simulink model "apartado233"  (Simulink 7.1)
settings: Solver=ode45  StartTime=0.0  StopTime=10000  RelTol=1e-3
undefined symbols (not defined in the file): p
libraries: simeventsrouting1 x15, simeventssink1 x13, simeventsattributes2 x6, simeventsqueue1 x6, simeventsgates1 x6, simeventsgenerators1 x6, simeventstiming1 x4, simeventsserver1 x3
settings Model: Creator=EmP  LastModifiedBy=EmP
settings SimEventsCC: propLogEventsScheduled=0  propLogEventsExecuted=0  propLogDepartureEvents=0  propDisplayEventCalendar=0  propDiagAttribOutput=1  propDiagFcnCallOutput=1  propDiagStatOutput=0

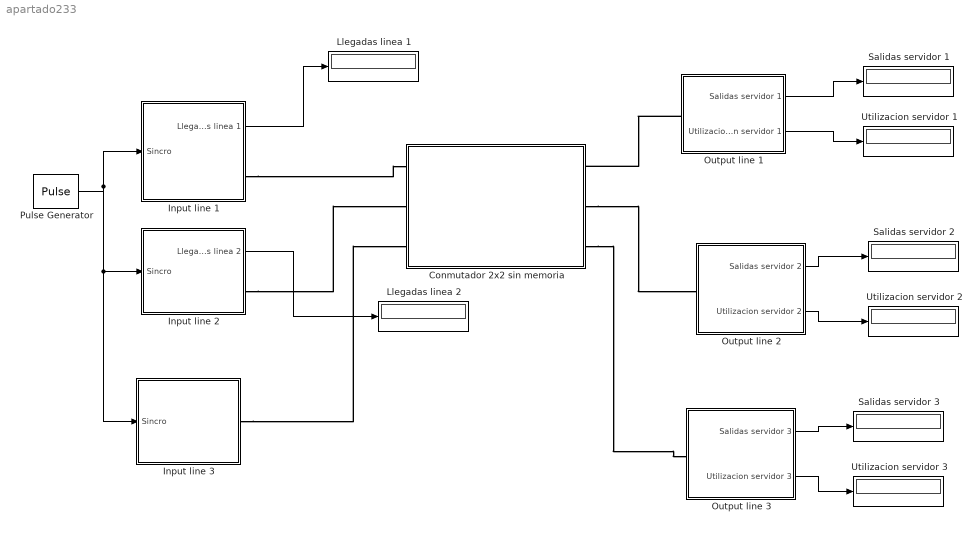
== system apartado233 ==
  Conmutador 2x2 sin memoria : Subsystem
  Input line 1 : Subsystem
  Input line 2 : Subsystem
  Input line 3 : Subsystem
  Llegadas linea 1 : Display
  Llegadas linea 2 : Display
  Output line 1 : Subsystem
  Output line 2 : Subsystem
  Output line 3 : Subsystem
  Pulse Generator : DiscretePulseGenerator  PulseType=Time based  Period=1  PulseWidth=50
  Salidas servidor 1 : Display
  Salidas servidor 2 : Display
  Salidas servidor 3 : Display
  Utilizacion servidor 1 : Display
  Utilizacion servidor 2 : Display
  Utilizacion servidor 3 : Display
  wires:
  Pulse Generator/1 -> Input line 1/1(Sincro), Input line 2/1(Sincro), Input line 3/1(Sincro)
  Input line 1/1(Llegadas linea 1) -> Llegadas linea 1/1
  Input line 2/1(Llegadas linea 2) -> Llegadas linea 2/1
  Output line 1/2(Utilizacion servidor 1) -> Utilizacion servidor 1/1
  Output line 1/1(Salidas servidor 1) -> Salidas servidor 1/1
  Output line 2/1(Salidas servidor 2) -> Salidas servidor 2/1
  Output line 2/2(Utilizacion servidor 2) -> Utilizacion servidor 2/1
  Output line 3/1(Salidas servidor 3) -> Salidas servidor 3/1
  Output line 3/2(Utilizacion servidor 3) -> Utilizacion servidor 3/1
  connections:
  Input line 1/RConn1 -- Conmutador 2x2 sin memoria/LConn1
  Input line 2/RConn1 -- Conmutador 2x2 sin memoria/LConn2
  Output line 1/LConn1 -- Conmutador 2x2 sin memoria/RConn1
  Conmutador 2x2 sin memoria/RConn2 -- Output line 2/LConn1
  Input line 3/RConn1 -- Conmutador 2x2 sin memoria/LConn3
  Conmutador 2x2 sin memoria/RConn3 -- Output line 3/LConn1

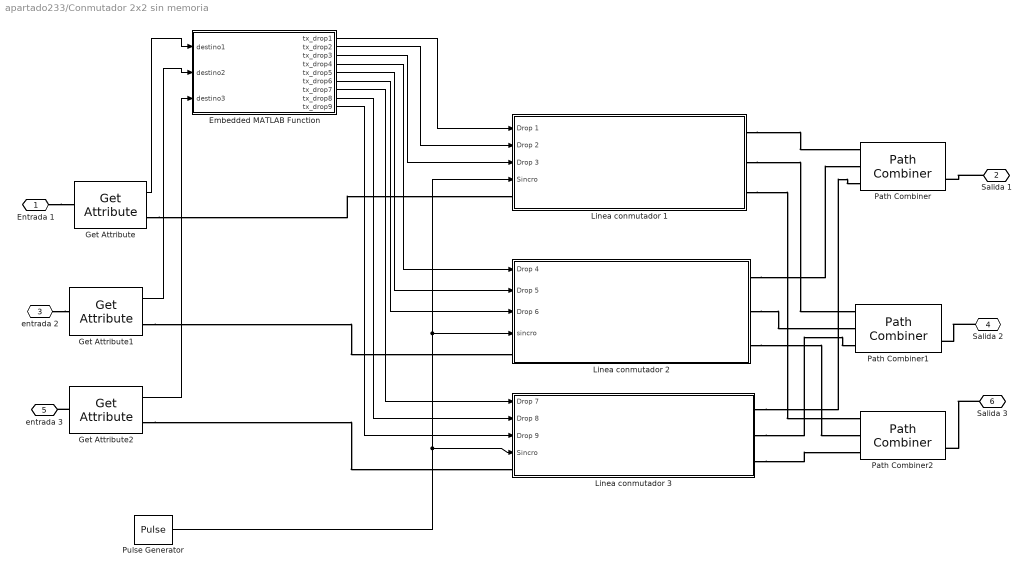
== system apartado233/Conmutador 2x2 sin memoria ==
  Embedded MATLAB Function : Stateflow chart
  Get Attribute : simeventsattributes2/Get Attribute  Priority=1  DialogController=des_ddg_create  DialogControllerArgs=DataTag1  SystemSampleTime=-1  AttributeName=Destino1  AttributeMissing=Error  AttributeDefaultValue=1  AttributeSendTiming=After entity departure  AttributeTreatAsVector=1  StatNumberDeparted=Off  EvaluatedDefaultAttributeValue={[]}
  Get Attribute1 : simeventsattributes2/Get Attribute  Priority=1  DialogController=des_ddg_create  DialogControllerArgs=DataTag3  SystemSampleTime=-1  AttributeName=Destino2  AttributeMissing=Error  AttributeDefaultValue=1  AttributeSendTiming=After entity departure  AttributeTreatAsVector=1  StatNumberDeparted=Off  EvaluatedDefaultAttributeValue={[]}
  Get Attribute2 : simeventsattributes2/Get Attribute  Priority=1  DialogController=des_ddg_create  DialogControllerArgs=DataTag5  SystemSampleTime=-1  AttributeName=Destino3  AttributeMissing=Error  AttributeDefaultValue=1  AttributeSendTiming=After entity departure  AttributeTreatAsVector=1  StatNumberDeparted=Off  EvaluatedDefaultAttributeValue={[]}
  Linea conmutador 1 : Subsystem
  Linea conmutador 2 : Subsystem
  Linea conmutador 3 : Subsystem
  Path Combiner : simeventsrouting1/Path Combiner  Priority=1  SystemSampleTime=-1  NumberInputPorts=3  InputPortPrecedence=IN1 port  InitialSeed=45675  SpecifyEventPriority=off  PriorityPathCombinerPortPrecedenceSelection=4100  StatNumberDeparted=On  StatLastArrivalPort=Off  EvaluatedNumPorts=3
  Path Combiner1 : simeventsrouting1/Path Combiner  Priority=1  SystemSampleTime=-1  NumberInputPorts=3  InputPortPrecedence=IN1 port  InitialSeed=45675  SpecifyEventPriority=off  PriorityPathCombinerPortPrecedenceSelection=4100  StatNumberDeparted=On  StatLastArrivalPort=Off  EvaluatedNumPorts=3
  Path Combiner2 : simeventsrouting1/Path Combiner  Priority=1  SystemSampleTime=-1  NumberInputPorts=3  InputPortPrecedence=IN1 port  InitialSeed=45675  SpecifyEventPriority=off  PriorityPathCombinerPortPrecedenceSelection=4100  StatNumberDeparted=On  StatLastArrivalPort=Off  EvaluatedNumPorts=3
  Pulse Generator : DiscretePulseGenerator  PulseType=Time based  Period=1  PulseWidth=50  PhaseDelay=0.5
  Entrada 1 : PMIOPort  Port=1  Side=Left
  Salida 1 : PMIOPort  Orientation=left  Port=2  Side=Right
  entrada 2 : PMIOPort  Port=3  Side=Left
  Salida 2 : PMIOPort  Orientation=left  Port=4  Side=Right
  entrada 3 : PMIOPort  Port=5  Side=Left
  Salida 3 : PMIOPort  Orientation=left  Port=6  Side=Right
  wires:
  Pulse Generator/1 -> Linea conmutador 3/4(Sincro), Linea conmutador 2/4(sincro), Linea conmutador 1/4(Sincro)
  Embedded MATLAB Function/1(tx_drop1) -> Linea conmutador 1/1(Drop 1)
  Embedded MATLAB Function/2(tx_drop2) -> Linea conmutador 1/2(Drop 2)
  Embedded MATLAB Function/3(tx_drop3) -> Linea conmutador 1/3(Drop 3)
  Embedded MATLAB Function/4(tx_drop4) -> Linea conmutador 2/1(Drop 4)
  Embedded MATLAB Function/5(tx_drop5) -> Linea conmutador 2/2(Drop 5)
  Embedded MATLAB Function/6(tx_drop6) -> Linea conmutador 2/3(Drop 6)
  Embedded MATLAB Function/7(tx_drop7) -> Linea conmutador 3/1(Drop 7)
  Embedded MATLAB Function/8(tx_drop8) -> Linea conmutador 3/2(Drop 8)
  Embedded MATLAB Function/9(tx_drop9) -> Linea conmutador 3/3(Drop 9)
  Get Attribute/1 -> Embedded MATLAB Function/1(destino1)
  Get Attribute1/1 -> Embedded MATLAB Function/2(destino2)
  Get Attribute2/1 -> Embedded MATLAB Function/3(destino3)
  connections:
  Entrada 1/RConn1 -- Get Attribute/LConn1
  Salida 1/RConn1 -- Path Combiner/RConn1
  entrada 2/RConn1 -- Get Attribute1/LConn1
  Salida 2/RConn1 -- Path Combiner1/RConn1
  Salida 3/RConn1 -- Path Combiner2/RConn1
  Get Attribute2/LConn1 -- entrada 3/RConn1
  Get Attribute/RConn1 -- Linea conmutador 1/LConn1
  Get Attribute1/RConn1 -- Linea conmutador 2/LConn1
  Get Attribute2/RConn1 -- Linea conmutador 3/LConn1
  Linea conmutador 1/RConn1 -- Path Combiner/LConn1
  Linea conmutador 1/RConn2 -- Path Combiner1/LConn1
  Linea conmutador 1/RConn3 -- Path Combiner2/LConn1
  Linea conmutador 2/RConn1 -- Path Combiner/LConn2
  Linea conmutador 2/RConn2 -- Path Combiner1/LConn2
  Linea conmutador 2/RConn3 -- Path Combiner2/LConn2
  Linea conmutador 3/RConn1 -- Path Combiner/LConn3
  Linea conmutador 3/RConn2 -- Path Combiner1/LConn3
  Linea conmutador 3/RConn3 -- Path Combiner2/LConn3

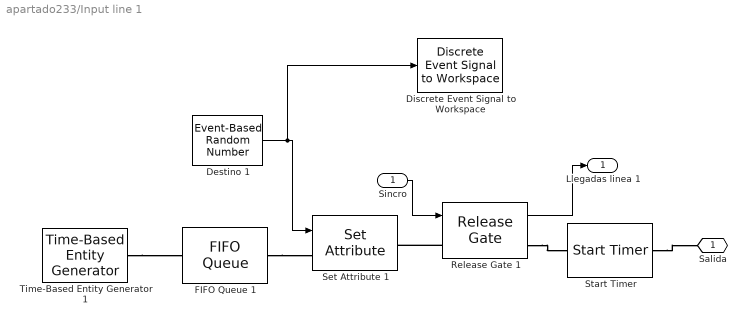
== system apartado233/Input line 1 ==
  Sincro : Inport
  Destino 1 : simeventsgenerators1/Signal Generators/Event-Based Random Number  SystemSampleTime=-1  distribution=Arbitrary discrete  meanExp=1  minUnif=1  maxUnif=2  pOneBern=0.25  pSuccessBino=0.5  numTrialBino=1  meanNorm=0  stdNorm=1  minTri=1  maxTri=3  modeTri=2  thresholdLogn=0  scaleLogn=1  shapeLogn=1  pSuccessGeo=0.5  meanPoiss=1  thresholdLogl=0  scaleLogl=1  thresholdGam=0  scaleGam=1  shapeGam=1  minBeta=0  maxBeta=1  shape1Beta=1  shape2Beta=1  minUnid=1  maxUnid=2  numValueUnid=2  thresholdWbl=0  scaleWbl=1  shapeWbl=1  valueVecCont=[0 1]  cdfVecCont=[0 1]  valueVecDisc=[0 1 2]  probVecDisc=[(1-p) p/2 p/2]  seed=875632  IsProcessed=on  isConnected=1
  Discrete Event Signal to Workspace : simeventssink1/Discrete Event Signal to Workspace  SystemSampleTime=-1  VariableName=destinoslinea1  SaveFormat=Array  IsMonitorOnly=off
  FIFO Queue 1 : simeventsqueue1/FIFO Queue  Priority=1  SystemSampleTime=-1  Capacity=inf  EnableTOPort=off  StatNumberDeparted=Off  StatNumberInBlock=Off  StatPendingEntity=Off  StatAverageWait=Off  StatAverageQueueLength=Off  StatNumberTimedout=Off
  Release Gate 1 : simeventsgates1/Release Gate  Priority=1  SystemSampleTime=-1  OpenGateUpon=Change in signal from port vc  SignalEdgeOption=Rising  SpecifyEventPriority=off  PriorityGateRelease=2200  StatNumberDeparted=On
  Set Attribute 1 : simeventsattributes2/Set Attribute  Priority=1  DialogController=des_ddg_create  DialogControllerArgs=DataTag39  SystemSampleTime=-1  AttributeFrom=Signal port  AttributeName=Destino1  AttributeTreatAsVector=1  AttributeValue=1  AttributeCreate=on  StatNumberDeparted=Off  EvaluatedAttributeValue={[]}
  Start Timer : simeventstiming1/Start Timer  Priority=0  SystemSampleTime=-1  TimerTag=retardo  TimerStartedOption=Warn and continue  StatNumberDeparted=Off
  Time-Based Entity Generator 1 : simeventsgenerators1/Entity Generators/Time-Based Entity Generator  Priority=1  DialogController=des_ddg_create  DialogControllerArgs=DataTag42  SystemSampleTime=-1  GenerateEntitiesUpon=Intergeneration time from dialog  Distribution=Constant  Minimum=0  Maximum=1  Mean=1  InitialSeed=12345  Period=0.5  PriorityEntityGeneration=300  GenerateEntityAtSimulationStart=on  ResponseWhenBlocked=Pause generation  ResponseWhenUnblocked=Immediate restart  EntityType=Blank  StatNumberDeparted=Off  StatPendingEntity=Off  StatAverageIntergenerationTime=Off
  Salida : PMIOPort  Orientation=left  Port=1  Side=Right
  Llegadas linea 1 : Outport  OutDataType=sfix(16)  OutScaling=2^0
  wires:
  Destino 1/1 -> Set Attribute 1/1, Discrete Event Signal to Workspace/1
  Sincro/1 -> Release Gate 1/1
  Release Gate 1/1 -> Llegadas linea 1/1
  connections:
  Time-Based Entity Generator 1/RConn1 -- FIFO Queue 1/LConn1
  FIFO Queue 1/RConn1 -- Set Attribute 1/LConn1
  Release Gate 1/LConn1 -- Set Attribute 1/RConn1
  Start Timer/RConn1 -- Salida/RConn1
  Release Gate 1/RConn1 -- Start Timer/LConn1

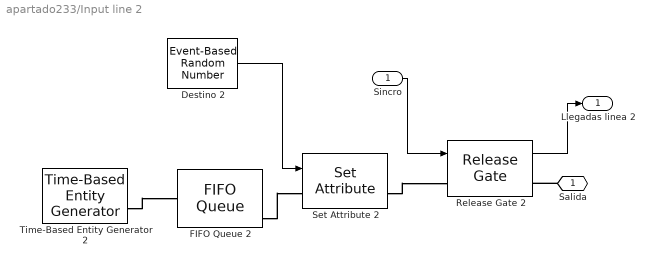
== system apartado233/Input line 2 ==
  Sincro : Inport
  Destino 2 : simeventsgenerators1/Signal Generators/Event-Based Random Number  SystemSampleTime=-1  distribution=Arbitrary discrete  meanExp=1  minUnif=1  maxUnif=1  pOneBern=0.25  pSuccessBino=0.5  numTrialBino=1  meanNorm=0  stdNorm=1  minTri=1  maxTri=3  modeTri=2  thresholdLogn=0  scaleLogn=1  shapeLogn=1  pSuccessGeo=0.5  meanPoiss=1  thresholdLogl=0  scaleLogl=1  thresholdGam=0  scaleGam=1  shapeGam=1  minBeta=0  maxBeta=1  shape1Beta=1  shape2Beta=1  minUnid=1  maxUnid=2  numValueUnid=2  thresholdWbl=0  scaleWbl=1  shapeWbl=1  valueVecCont=[0 1]  cdfVecCont=[0 1]  valueVecDisc=[0 1 2]  probVecDisc=[(1-p) p/2 p/2]  seed=0964  IsProcessed=on  isConnected=1
  FIFO Queue 2 : simeventsqueue1/FIFO Queue  Priority=1  SystemSampleTime=-1  Capacity=1000000  EnableTOPort=off  StatNumberDeparted=On  StatNumberInBlock=On  StatPendingEntity=Off  StatAverageWait=Off  StatAverageQueueLength=Off  StatNumberTimedout=Off
  Release Gate 2 : simeventsgates1/Release Gate  Priority=1  SystemSampleTime=-1  OpenGateUpon=Change in signal from port vc  SignalEdgeOption=Rising  SpecifyEventPriority=off  PriorityGateRelease=2200  StatNumberDeparted=On
  Set Attribute 2 : simeventsattributes2/Set Attribute  Priority=1  DialogController=des_ddg_create  DialogControllerArgs=DataTag46  SystemSampleTime=-1  AttributeFrom=Signal port  AttributeName=Destino2  AttributeTreatAsVector=1  AttributeValue=1  AttributeCreate=on  StatNumberDeparted=On  EvaluatedAttributeValue={[]}
  Time-Based Entity Generator 2 : simeventsgenerators1/Entity Generators/Time-Based Entity Generator  Priority=1  DialogController=des_ddg_create  DialogControllerArgs=DataTag48  SystemSampleTime=-1  GenerateEntitiesUpon=Intergeneration time from dialog  Distribution=Constant  Minimum=0  Maximum=1  Mean=1  InitialSeed=543541  Period=1  PriorityEntityGeneration=300  GenerateEntityAtSimulationStart=on  ResponseWhenBlocked=Pause generation  ResponseWhenUnblocked=Immediate restart  EntityType=Blank  StatNumberDeparted=On  StatPendingEntity=Off  StatAverageIntergenerationTime=Off
  Salida : PMIOPort  Orientation=left  Port=1  Side=Right
  Llegadas linea 2 : Outport  OutDataType=sfix(16)  OutScaling=2^0
  wires:
  Destino 2/1 -> Set Attribute 2/1
  Sincro/1 -> Release Gate 2/1
  Release Gate 2/1 -> Llegadas linea 2/1
  connections:
  Time-Based Entity Generator 2/RConn1 -- FIFO Queue 2/LConn1
  FIFO Queue 2/RConn1 -- Set Attribute 2/LConn1
  Set Attribute 2/RConn1 -- Release Gate 2/LConn1
  Salida/RConn1 -- Release Gate 2/RConn1

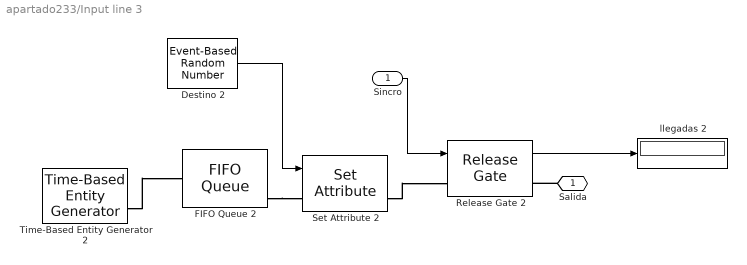
== system apartado233/Input line 3 ==
  Sincro : Inport
  Destino 2 : simeventsgenerators1/Signal Generators/Event-Based Random Number  SystemSampleTime=-1  distribution=Arbitrary discrete  meanExp=1  minUnif=1  maxUnif=1  pOneBern=0.25  pSuccessBino=0.5  numTrialBino=1  meanNorm=0  stdNorm=1  minTri=1  maxTri=3  modeTri=2  thresholdLogn=0  scaleLogn=1  shapeLogn=1  pSuccessGeo=0.5  meanPoiss=1  thresholdLogl=0  scaleLogl=1  thresholdGam=0  scaleGam=1  shapeGam=1  minBeta=0  maxBeta=1  shape1Beta=1  shape2Beta=1  minUnid=1  maxUnid=2  numValueUnid=2  thresholdWbl=0  scaleWbl=1  shapeWbl=1  valueVecCont=[0 1]  cdfVecCont=[0 1]  valueVecDisc=[0 1 2]  probVecDisc=[(1-p) p/2 p/2]  seed=45287634  IsProcessed=on  isConnected=1
  FIFO Queue 2 : simeventsqueue1/FIFO Queue  Priority=1  SystemSampleTime=-1  Capacity=1000000  EnableTOPort=off  StatNumberDeparted=On  StatNumberInBlock=On  StatPendingEntity=Off  StatAverageWait=Off  StatAverageQueueLength=Off  StatNumberTimedout=Off
  Release Gate 2 : simeventsgates1/Release Gate  Priority=1  SystemSampleTime=-1  OpenGateUpon=Change in signal from port vc  SignalEdgeOption=Rising  SpecifyEventPriority=off  PriorityGateRelease=2200  StatNumberDeparted=On
  Set Attribute 2 : simeventsattributes2/Set Attribute  Priority=1  DialogController=des_ddg_create  DialogControllerArgs=DataTag52  SystemSampleTime=-1  AttributeFrom=Signal port  AttributeName=Destino3  AttributeTreatAsVector=1  AttributeValue=1  AttributeCreate=on  StatNumberDeparted=On  EvaluatedAttributeValue={[]}
  Time-Based Entity Generator 2 : simeventsgenerators1/Entity Generators/Time-Based Entity Generator  Priority=1  DialogController=des_ddg_create  DialogControllerArgs=DataTag54  SystemSampleTime=-1  GenerateEntitiesUpon=Intergeneration time from dialog  Distribution=Constant  Minimum=0  Maximum=1  Mean=1  InitialSeed=543541  Period=1  PriorityEntityGeneration=300  GenerateEntityAtSimulationStart=on  ResponseWhenBlocked=Pause generation  ResponseWhenUnblocked=Immediate restart  EntityType=Blank  StatNumberDeparted=On  StatPendingEntity=Off  StatAverageIntergenerationTime=Off
  llegadas 2 : Display
  Salida : PMIOPort  Orientation=left  Port=1  Side=Right
  wires:
  Destino 2/1 -> Set Attribute 2/1
  Sincro/1 -> Release Gate 2/1
  Release Gate 2/1 -> llegadas 2/1
  connections:
  Time-Based Entity Generator 2/RConn1 -- FIFO Queue 2/LConn1
  FIFO Queue 2/RConn1 -- Set Attribute 2/LConn1
  Set Attribute 2/RConn1 -- Release Gate 2/LConn1
  Salida/RConn1 -- Release Gate 2/RConn1

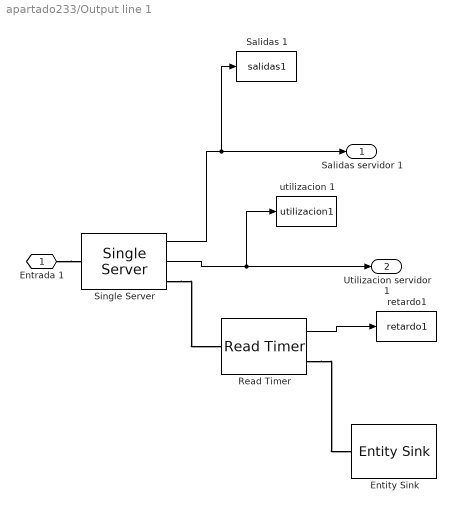
== system apartado233/Output line 1 ==
  Entity Sink : simeventssink1/Entity Sink  Priority=1  SystemSampleTime=-1  AvailableForArrivals=on  StatNumberArrived=Off
  Read Timer : simeventstiming1/Read Timer  Priority=0  SystemSampleTime=-1  TimerTag=retardo  TimerModeOption=Ignore  TimerStop=off  StatNumberDeparted=Off  StatTimerNumberDeparted=Off  StatTimeElapsed=Off  StatAverageTimeElapsed=On
  Salidas 1 : ToWorkspace  VariableName=salidas1  SampleTime=10000  SaveFormat=Array
  Single Server : simeventsserver1/Single Server  Priority=1  SystemSampleTime=-1  ServiceTimeFrom=Dialog  ServiceTime=0.99999  AttributeName=ServiceTime  PriorityServiceCompletion=500  PermitPreemption=off  SortingAttributeName=PriorityAttributeName  SortingDirection=Ascending  WriteToAttribute=off  ResidualAttributeName=ResidualServiceTime  CreateAttribute=on  EnableTOPort=off  StatNumberDeparted=On  StatNumberInBlock=Off  StatNumberPreempted=Off  StatPendingEntity=Off  StatAverageWait=Off  StatUtilization=On  StatNumberTimedout=Off
  retardo1 : ToWorkspace  VariableName=retardo1  SampleTime=10000  SaveFormat=Array
  utilizacion 1 : ToWorkspace  VariableName=utilizacion1  SampleTime=10000  SaveFormat=Array
  Entrada 1 : PMIOPort  Port=1  Side=Left
  Salidas servidor 1 : Outport  OutDataType=sfix(16)  OutScaling=2^0
  Utilizacion servidor 1 : Outport  Port=2  OutDataType=sfix(16)  OutScaling=2^0
  wires:
  Single Server/1 -> Salidas 1/1, Salidas servidor 1/1
  Single Server/2 -> Utilizacion servidor 1/1, utilizacion 1/1
  Read Timer/1 -> retardo1/1
  connections:
  Entrada 1/RConn1 -- Single Server/LConn1
  Read Timer/RConn1 -- Entity Sink/LConn1
  Single Server/RConn1 -- Read Timer/LConn1

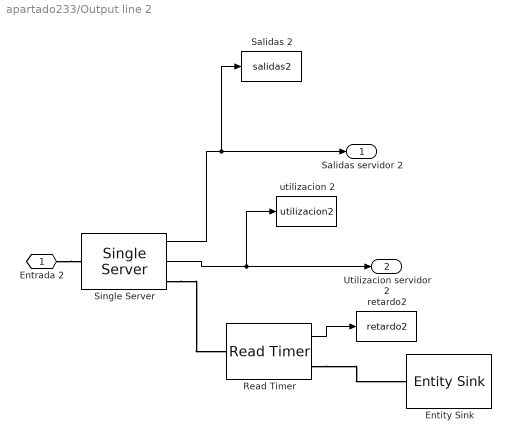
== system apartado233/Output line 2 ==
  Entity Sink : simeventssink1/Entity Sink  Priority=1  SystemSampleTime=-1  AvailableForArrivals=on  StatNumberArrived=Off
  Read Timer : simeventstiming1/Read Timer  Priority=0  SystemSampleTime=-1  TimerTag=retardo  TimerModeOption=Ignore  TimerStop=off  StatNumberDeparted=Off  StatTimerNumberDeparted=Off  StatTimeElapsed=Off  StatAverageTimeElapsed=On
  Salidas 2 : ToWorkspace  VariableName=salidas2  SampleTime=10000  SaveFormat=Array
  Single Server : simeventsserver1/Single Server  Priority=1  SystemSampleTime=-1  ServiceTimeFrom=Dialog  ServiceTime=0.99999  AttributeName=ServiceTime  PriorityServiceCompletion=500  PermitPreemption=off  SortingAttributeName=PriorityAttributeName  SortingDirection=Ascending  WriteToAttribute=off  ResidualAttributeName=ResidualServiceTime  CreateAttribute=on  EnableTOPort=off  StatNumberDeparted=On  StatNumberInBlock=Off  StatNumberPreempted=Off  StatPendingEntity=Off  StatAverageWait=Off  StatUtilization=On  StatNumberTimedout=Off
  retardo2 : ToWorkspace  VariableName=retardo2  SampleTime=10000  SaveFormat=Array
  utilizacion 2 : ToWorkspace  VariableName=utilizacion2  SampleTime=10000  SaveFormat=Array
  Entrada 2 : PMIOPort  Port=1  Side=Left
  Salidas servidor 2 : Outport  OutDataType=sfix(16)  OutScaling=2^0
  Utilizacion servidor 2 : Outport  Port=2  OutDataType=sfix(16)  OutScaling=2^0
  wires:
  Single Server/1 -> Salidas 2/1, Salidas servidor 2/1
  Single Server/2 -> Utilizacion servidor 2/1, utilizacion 2/1
  Read Timer/1 -> retardo2/1
  connections:
  Entrada 2/RConn1 -- Single Server/LConn1
  Read Timer/RConn1 -- Entity Sink/LConn1
  Single Server/RConn1 -- Read Timer/LConn1

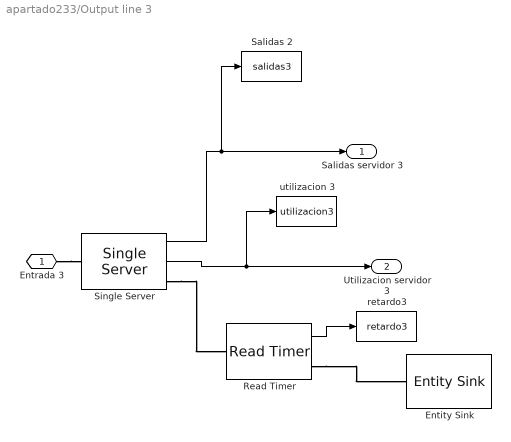
== system apartado233/Output line 3 ==
  Entity Sink : simeventssink1/Entity Sink  Priority=1  SystemSampleTime=-1  AvailableForArrivals=on  StatNumberArrived=Off
  Read Timer : simeventstiming1/Read Timer  Priority=0  SystemSampleTime=-1  TimerTag=retardo  TimerModeOption=Ignore  TimerStop=off  StatNumberDeparted=Off  StatTimerNumberDeparted=Off  StatTimeElapsed=Off  StatAverageTimeElapsed=On
  Salidas 2 : ToWorkspace  VariableName=salidas3  SampleTime=10000  SaveFormat=Array
  Single Server : simeventsserver1/Single Server  Priority=1  SystemSampleTime=-1  ServiceTimeFrom=Dialog  ServiceTime=0.99999  AttributeName=ServiceTime  PriorityServiceCompletion=500  PermitPreemption=off  SortingAttributeName=PriorityAttributeName  SortingDirection=Ascending  WriteToAttribute=off  ResidualAttributeName=ResidualServiceTime  CreateAttribute=on  EnableTOPort=off  StatNumberDeparted=On  StatNumberInBlock=Off  StatNumberPreempted=Off  StatPendingEntity=Off  StatAverageWait=Off  StatUtilization=On  StatNumberTimedout=Off
  retardo3 : ToWorkspace  VariableName=retardo3  SampleTime=10000  SaveFormat=Array
  utilizacion 3 : ToWorkspace  VariableName=utilizacion3  SampleTime=10000  SaveFormat=Array
  Entrada 3 : PMIOPort  Port=1  Side=Left
  Salidas servidor 3 : Outport  OutDataType=sfix(16)  OutScaling=2^0
  Utilizacion servidor 3 : Outport  Port=2  OutDataType=sfix(16)  OutScaling=2^0
  wires:
  Single Server/1 -> Salidas 2/1, Salidas servidor 3/1
  Single Server/2 -> Utilizacion servidor 3/1, utilizacion 3/1
  Read Timer/1 -> retardo3/1
  connections:
  Entrada 3/RConn1 -- Single Server/LConn1
  Read Timer/RConn1 -- Entity Sink/LConn1
  Single Server/RConn1 -- Read Timer/LConn1

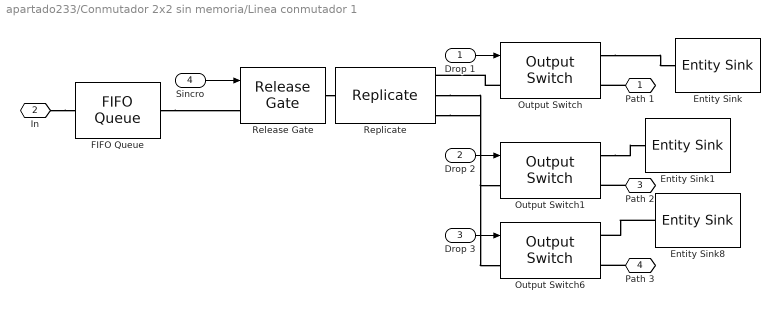
== system apartado233/Conmutador 2x2 sin memoria/Linea conmutador 1 ==
  Drop 1 : Inport
  Drop 2 : Inport  Port=2
  Drop 3 : Inport  Port=3
  Sincro : Inport  Port=4
  Entity Sink : simeventssink1/Entity Sink  Priority=1  SystemSampleTime=-1  AvailableForArrivals=on  StatNumberArrived=Off
  Entity Sink1 : simeventssink1/Entity Sink  Priority=1  SystemSampleTime=-1  AvailableForArrivals=on  StatNumberArrived=Off
  Entity Sink8 : simeventssink1/Entity Sink  Priority=1  SystemSampleTime=-1  AvailableForArrivals=on  StatNumberArrived=Off
  FIFO Queue : simeventsqueue1/FIFO Queue  Priority=1  SystemSampleTime=-1  Capacity=1  EnableTOPort=off  StatNumberDeparted=Off  StatNumberInBlock=Off  StatPendingEntity=Off  StatAverageWait=Off  StatAverageQueueLength=Off  StatNumberTimedout=Off
  Output Switch : simeventsrouting1/Output Switch  Priority=1  SystemSampleTime=-1  NumberOutputPorts=2  SwitchingCriterion=From signal port p  InitialSeed=34567  AttributeName=Attribute1  InitialConditionsOpt=off  InitialConditions=1  EntityBufferOpt=off  SpecifyEventPriority=off  PriorityOutputSwitchSelectPort=4100  TimeoutPortOpt=off  StatNumberDeparted=Off  StatNumberTimedOut=Off  StatPendingEntity=Off  StatLastDeparturePort=Off  EvaluatedNumPorts=2
  Output Switch1 : simeventsrouting1/Output Switch  Priority=1  SystemSampleTime=-1  NumberOutputPorts=2  SwitchingCriterion=From signal port p  InitialSeed=34567  AttributeName=Attribute1  InitialConditionsOpt=off  InitialConditions=1  EntityBufferOpt=off  SpecifyEventPriority=off  PriorityOutputSwitchSelectPort=4100  TimeoutPortOpt=off  StatNumberDeparted=Off  StatNumberTimedOut=Off  StatPendingEntity=Off  StatLastDeparturePort=Off  EvaluatedNumPorts=2
  Output Switch6 : simeventsrouting1/Output Switch  Priority=1  SystemSampleTime=-1  NumberOutputPorts=2  SwitchingCriterion=From signal port p  InitialSeed=34567  AttributeName=Attribute1  InitialConditionsOpt=off  InitialConditions=1  EntityBufferOpt=off  SpecifyEventPriority=off  PriorityOutputSwitchSelectPort=4100  TimeoutPortOpt=off  StatNumberDeparted=Off  StatNumberTimedOut=Off  StatPendingEntity=Off  StatLastDeparturePort=Off  EvaluatedNumPorts=2
  Release Gate : simeventsgates1/Release Gate  Priority=1  SystemSampleTime=-1  OpenGateUpon=Change in signal from port vc  SignalEdgeOption=Rising  SpecifyEventPriority=off  PriorityGateRelease=2200  StatNumberDeparted=Off
  Replicate : simeventsrouting1/Replicate  Priority=1  SystemSampleTime=-1  NumberOutputPorts=3  ReplicateEntityWhen=All entity output ports are not blocked  OutputPortPrecedence=OUT1 port  InitialSeed=56789  ActionUponBlocking=Discard entity  StatNumberArrived=Off  StatNumberDeparted=Off  EvaluatedNumPorts=3
  Path 1 : PMIOPort  Orientation=left  Port=1  Side=Right
  In : PMIOPort  Port=2  Side=Left
  Path 2 : PMIOPort  Orientation=left  Port=3  Side=Right
  Path 3 : PMIOPort  Orientation=left  Port=4  Side=Right
  wires:
  Sincro/1 -> Release Gate/1
  Drop 1/1 -> Output Switch/1
  Drop 2/1 -> Output Switch1/1
  Drop 3/1 -> Output Switch6/1
  connections:
  Output Switch/RConn1 -- Entity Sink/LConn1
  Output Switch1/RConn1 -- Entity Sink1/LConn1
  Entity Sink8/LConn1 -- Output Switch6/RConn1
  FIFO Queue/RConn1 -- Release Gate/LConn1
  Output Switch/LConn1 -- Replicate/RConn1
  Replicate/RConn2 -- Output Switch1/LConn1
  Replicate/RConn3 -- Output Switch6/LConn1
  Release Gate/RConn1 -- Replicate/LConn1
  Path 1/RConn1 -- Output Switch/RConn2
  In/RConn1 -- FIFO Queue/LConn1
  Path 2/RConn1 -- Output Switch1/RConn2
  Path 3/RConn1 -- Output Switch6/RConn2

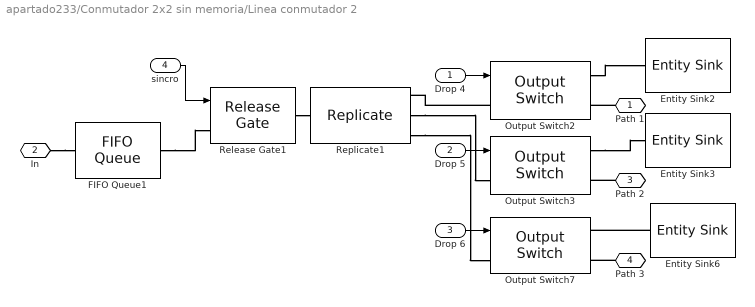
== system apartado233/Conmutador 2x2 sin memoria/Linea conmutador 2 ==
  Drop 4 : Inport
  Drop 5 : Inport  Port=2
  Drop 6 : Inport  Port=3
  sincro : Inport  Port=4
  Entity Sink2 : simeventssink1/Entity Sink  Priority=1  SystemSampleTime=-1  AvailableForArrivals=on  StatNumberArrived=Off
  Entity Sink3 : simeventssink1/Entity Sink  Priority=1  SystemSampleTime=-1  AvailableForArrivals=on  StatNumberArrived=Off
  Entity Sink6 : simeventssink1/Entity Sink  Priority=1  SystemSampleTime=-1  AvailableForArrivals=on  StatNumberArrived=Off
  FIFO Queue1 : simeventsqueue1/FIFO Queue  Priority=1  SystemSampleTime=-1  Capacity=1  EnableTOPort=off  StatNumberDeparted=Off  StatNumberInBlock=Off  StatPendingEntity=Off  StatAverageWait=Off  StatAverageQueueLength=Off  StatNumberTimedout=Off
  Output Switch2 : simeventsrouting1/Output Switch  Priority=1  SystemSampleTime=-1  NumberOutputPorts=2  SwitchingCriterion=From signal port p  InitialSeed=34567  AttributeName=Attribute1  InitialConditionsOpt=off  InitialConditions=1  EntityBufferOpt=off  SpecifyEventPriority=off  PriorityOutputSwitchSelectPort=4100  TimeoutPortOpt=off  StatNumberDeparted=Off  StatNumberTimedOut=Off  StatPendingEntity=Off  StatLastDeparturePort=Off  EvaluatedNumPorts=2
  Output Switch3 : simeventsrouting1/Output Switch  Priority=1  SystemSampleTime=-1  NumberOutputPorts=2  SwitchingCriterion=From signal port p  InitialSeed=34567  AttributeName=Attribute1  InitialConditionsOpt=off  InitialConditions=1  EntityBufferOpt=off  SpecifyEventPriority=off  PriorityOutputSwitchSelectPort=4100  TimeoutPortOpt=off  StatNumberDeparted=Off  StatNumberTimedOut=Off  StatPendingEntity=Off  StatLastDeparturePort=Off  EvaluatedNumPorts=2
  Output Switch7 : simeventsrouting1/Output Switch  Priority=1  SystemSampleTime=-1  NumberOutputPorts=2  SwitchingCriterion=From signal port p  InitialSeed=34567  AttributeName=Attribute1  InitialConditionsOpt=off  InitialConditions=1  EntityBufferOpt=off  SpecifyEventPriority=off  PriorityOutputSwitchSelectPort=4100  TimeoutPortOpt=off  StatNumberDeparted=Off  StatNumberTimedOut=Off  StatPendingEntity=Off  StatLastDeparturePort=Off  EvaluatedNumPorts=2
  Release Gate1 : simeventsgates1/Release Gate  Priority=1  SystemSampleTime=-1  OpenGateUpon=Change in signal from port vc  SignalEdgeOption=Rising  SpecifyEventPriority=off  PriorityGateRelease=2200  StatNumberDeparted=Off
  Replicate1 : simeventsrouting1/Replicate  Priority=1  SystemSampleTime=-1  NumberOutputPorts=3  ReplicateEntityWhen=All entity output ports are not blocked  OutputPortPrecedence=OUT1 port  InitialSeed=56789  ActionUponBlocking=Discard entity  StatNumberArrived=Off  StatNumberDeparted=Off  EvaluatedNumPorts=3
  Path 1 : PMIOPort  Orientation=left  Port=1  Side=Right
  In : PMIOPort  Port=2  Side=Left
  Path 2 : PMIOPort  Orientation=left  Port=3  Side=Right
  Path 3 : PMIOPort  Orientation=left  Port=4  Side=Right
  wires:
  sincro/1 -> Release Gate1/1
  Drop 4/1 -> Output Switch2/1
  Drop 5/1 -> Output Switch3/1
  Drop 6/1 -> Output Switch7/1
  connections:
  Output Switch2/RConn1 -- Entity Sink2/LConn1
  Output Switch3/RConn1 -- Entity Sink3/LConn1
  Entity Sink6/LConn1 -- Output Switch7/RConn1
  FIFO Queue1/RConn1 -- Release Gate1/LConn1
  Output Switch2/LConn1 -- Replicate1/RConn1
  Replicate1/RConn2 -- Output Switch3/LConn1
  Replicate1/RConn3 -- Output Switch7/LConn1
  Release Gate1/RConn1 -- Replicate1/LConn1
  Path 1/RConn1 -- Output Switch2/RConn2
  In/RConn1 -- FIFO Queue1/LConn1
  Path 2/RConn1 -- Output Switch3/RConn2
  Path 3/RConn1 -- Output Switch7/RConn2

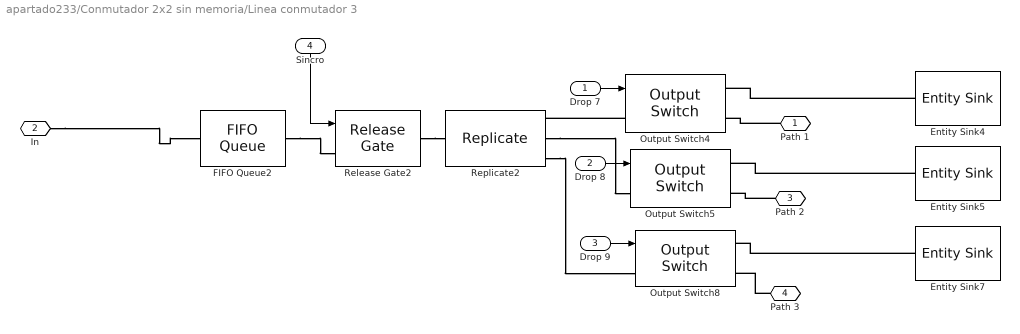
== system apartado233/Conmutador 2x2 sin memoria/Linea conmutador 3 ==
  Drop 7 : Inport
  Drop 8 : Inport  Port=2
  Drop 9 : Inport  Port=3
  Sincro : Inport  Orientation=down  Port=4
  Entity Sink4 : simeventssink1/Entity Sink  Priority=1  SystemSampleTime=-1  AvailableForArrivals=on  StatNumberArrived=Off
  Entity Sink5 : simeventssink1/Entity Sink  Priority=1  SystemSampleTime=-1  AvailableForArrivals=on  StatNumberArrived=Off
  Entity Sink7 : simeventssink1/Entity Sink  Priority=1  SystemSampleTime=-1  AvailableForArrivals=on  StatNumberArrived=Off
  FIFO Queue2 : simeventsqueue1/FIFO Queue  Priority=1  SystemSampleTime=-1  Capacity=1  EnableTOPort=off  StatNumberDeparted=Off  StatNumberInBlock=Off  StatPendingEntity=Off  StatAverageWait=Off  StatAverageQueueLength=Off  StatNumberTimedout=Off
  Output Switch4 : simeventsrouting1/Output Switch  Priority=1  SystemSampleTime=-1  NumberOutputPorts=2  SwitchingCriterion=From signal port p  InitialSeed=34567  AttributeName=Attribute1  InitialConditionsOpt=off  InitialConditions=1  EntityBufferOpt=off  SpecifyEventPriority=off  PriorityOutputSwitchSelectPort=4100  TimeoutPortOpt=off  StatNumberDeparted=Off  StatNumberTimedOut=Off  StatPendingEntity=Off  StatLastDeparturePort=Off  EvaluatedNumPorts=2
  Output Switch5 : simeventsrouting1/Output Switch  Priority=1  SystemSampleTime=-1  NumberOutputPorts=2  SwitchingCriterion=From signal port p  InitialSeed=34567  AttributeName=Attribute1  InitialConditionsOpt=off  InitialConditions=1  EntityBufferOpt=off  SpecifyEventPriority=off  PriorityOutputSwitchSelectPort=4100  TimeoutPortOpt=off  StatNumberDeparted=Off  StatNumberTimedOut=Off  StatPendingEntity=Off  StatLastDeparturePort=Off  EvaluatedNumPorts=2
  Output Switch8 : simeventsrouting1/Output Switch  Priority=1  SystemSampleTime=-1  NumberOutputPorts=2  SwitchingCriterion=From signal port p  InitialSeed=34567  AttributeName=Attribute1  InitialConditionsOpt=off  InitialConditions=1  EntityBufferOpt=off  SpecifyEventPriority=off  PriorityOutputSwitchSelectPort=4100  TimeoutPortOpt=off  StatNumberDeparted=Off  StatNumberTimedOut=Off  StatPendingEntity=Off  StatLastDeparturePort=Off  EvaluatedNumPorts=2
  Release Gate2 : simeventsgates1/Release Gate  Priority=1  SystemSampleTime=-1  OpenGateUpon=Change in signal from port vc  SignalEdgeOption=Rising  SpecifyEventPriority=off  PriorityGateRelease=2200  StatNumberDeparted=Off
  Replicate2 : simeventsrouting1/Replicate  Priority=1  SystemSampleTime=-1  NumberOutputPorts=3  ReplicateEntityWhen=All entity output ports are not blocked  OutputPortPrecedence=OUT1 port  InitialSeed=56789  ActionUponBlocking=Discard entity  StatNumberArrived=Off  StatNumberDeparted=Off  EvaluatedNumPorts=3
  Path 1 : PMIOPort  Orientation=left  Port=1  Side=Right
  In : PMIOPort  Port=2  Side=Left
  Path 2 : PMIOPort  Orientation=left  Port=3  Side=Right
  Path 3 : PMIOPort  Orientation=left  Port=4  Side=Right
  wires:
  Sincro/1 -> Release Gate2/1
  Drop 7/1 -> Output Switch4/1
  Drop 8/1 -> Output Switch5/1
  Drop 9/1 -> Output Switch8/1
  connections:
  Entity Sink4/LConn1 -- Output Switch4/RConn1
  Entity Sink5/LConn1 -- Output Switch5/RConn1
  Entity Sink7/LConn1 -- Output Switch8/RConn1
  FIFO Queue2/RConn1 -- Release Gate2/LConn1
  Output Switch4/LConn1 -- Replicate2/RConn1
  Replicate2/RConn2 -- Output Switch5/LConn1
  Replicate2/RConn3 -- Output Switch8/LConn1
  Release Gate2/RConn1 -- Replicate2/LConn1
  Path 1/RConn1 -- Output Switch4/RConn2
  In/RConn1 -- FIFO Queue2/LConn1
  Path 2/RConn1 -- Output Switch5/RConn2
  Path 3/RConn1 -- Output Switch8/RConn2

== matlab function Conmutador 2x2 sin memoria/Embedded MATLAB Function ==
  data: destino1 input double; tx_drop1 output double; destino2 input double; tx_drop2 output double; tx_drop3 output double; tx_drop4 output double; destino3 input double; tx_drop5 output double; tx_drop6 output double; tx_drop7 output double; tx_drop8 output double; tx_drop9 output double
function [tx_drop1, tx_drop2,tx_drop3,tx_drop4, tx_drop5, tx_drop6, tx_drop7, tx_drop8, tx_drop9] = port_selection_line(destino1,destino2,destino3)

%matriz de puertos de salida:(filas=entradas, columnas=salidas) Inicialmente todos los paquetes se descartan
puertos_salida=ones(2,2);           %en el modelo si el puerto de salida tiene valor 1, el paquete de tira
%vector de destinos de cada entrada
%la posicion del vector corresponde a la linea de entrada y el valor corresponde a la linea de destino
%exactamente, los destinos representan las lineas de salida, que no son lo mismo que los puertos de salida.
%los puertos de salida se asocian con cada linea de salida segun esta implementado el modelo de simulink
destinos=[destino1, destino2];      

%%%%%%%Configurar la matriz de conmutacion con las asociaciones correspondientes %%%%%%%

for i=1:1:length(destinos)
      puertos_salida(i,:)=designar_puertos(destinos(i));       %llamamos a la funcion que asocia un destino con los puertos de salida
end

%%%%%% Analizar las columnas de la matriz para ver si existen colisiones %%%%%%%
%comprobamos que en una misma columna de la matriz de puertos de salida no haya mas de un elemento distinto de 1,
%ya que en ese caso, hay dos paquetes que quieren ir la misma linea de salida (mismo destino)
for i=1:length(puertos_salida(1,:))
     entradas_en_conflicto=zeros(1,length(destinos));          %este vector contiene las entradas que colisionan
     %comprobamos si se repite la misma salida 
     for j=1:length(puertos_salida(:,1))
        
         if puertos_salida(j,i)==2
            entradas_en_conflicto(j)=1;                     %con esto indicamos que la entrada j quiere salir por la linea 1
         end    
     end    %end for j

     %ahora vemos si se han producido colisiones y si es asi resolvemos el conflicto
     if sum(entradas_en_conflicto)>1                         %si mas de una entrada sale por el mismo sitio
        entrada=elegir_entrada(entradas_en_conflicto) ;       %seleccionamos cual de ellas es la que finalmente alcanza su destino
        puertos_salida(:,i)=resolver_conflicto(entrada);        %modificamos la matriz de puertos de salida con la asociacion correspondiente
     end
end %end for i

%%%%%% Crear las asociaciones entre la matriz de conmutacion y las lineas de salida %%%%%%%%%%% 
tx_drop1=puertos_salida(1,1);
tx_drop2=puertos_salida(1,2);
tx_drop3=puertos_salida(2,1);
tx_drop4=puertos_salida(2,2);

%%%%%% Funcion que asocia una salida con la configuracion de los puertos de salida correspondiente. %%%%%%
% si el elemento i,j vale 2 es que la entrada i quiere salir por la salida j
function [puertos]=designar_puertos(destino)
    puertos=ones(1,2);
    if destino~=0
        puertos(destino)=2;
    end

%%%%%%%%% Funcion que escoge un elemento entre N elementos al azar %%%%%%%%%
% N viene determinado por la suma de los elementos del vector entradas
%entradas contiene que lineas de entrada han colisionado
%la funcion escoge una linea de entre todas las que colisionan
function [ent]=elegir_entrada(entradas)
    cont=0;
    ent=0;
    aux=sum(entradas);
    seleccion=ceil(aux.*rand(1));
    for i=1:length(entradas)
     
        if entradas(i)==1
            cont=cont+1;
            if cont==seleccion
            ent=i;
            end
        end
    end
    
%%%%% Funcion que asigna los puertos de salida segun la entrada %%%%%%%
%esta asignacion se hace por columnas, de forma que soluciona las posibles colisiones
%toda la columna vale 1 excepto la posicion indicada por entrada
function [columna]=resolver_conflicto(entrada)
    columna=ones(2,1);
    columna(entrada)=2;
